simulink model "sxem_79"  (R2023a)
settings: Solver=VariableStepAuto  StartTime=0.0  StopTime=40.0  RelTol=1e-3
settings Model: Creator=User  LastModifiedBy=User

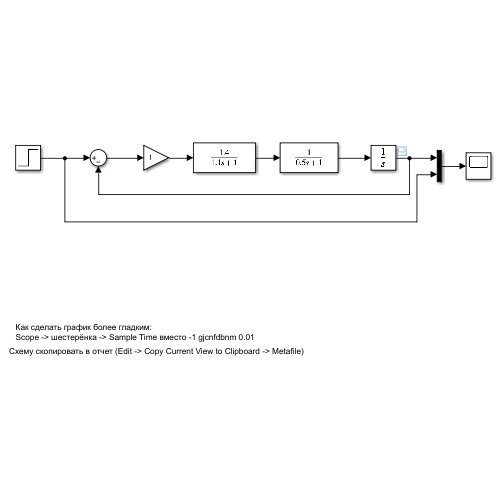
[thumbnail: Simulink's stored preview of the top-level diagram]
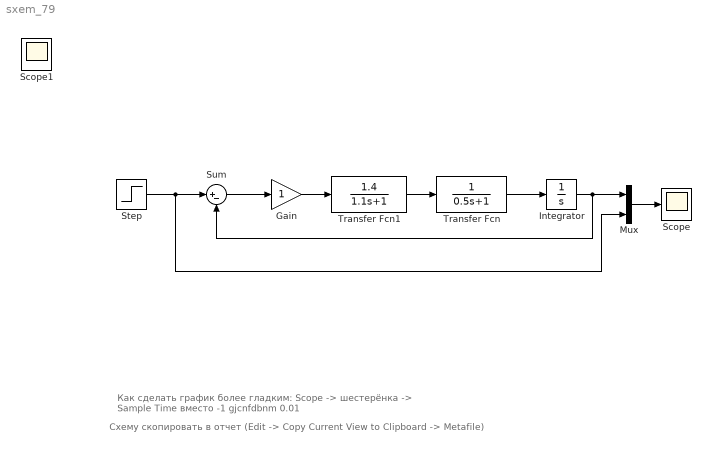
== system sxem_79 ==
  note: Как сделать график более гладким:
      | Scope -> шестерёнка -> Sample Time вместо -1 gjcnfdbnm 0.01
  note: Схему скопировать в отчет (Edit -> Copy Current View to Clipboard -> Metafile)
  Gain : Gain
  Integrator : Integrator
  Mux : Mux  Inputs=2
  Scope : Scope
  Step : Step  Time=0  SampleTime=0
  Sum : Sum  Inputs=|+-
  Transfer Fcn : TransferFcn  Denominator=[0.5 1]
  Transfer Fcn1 : TransferFcn  Numerator=[1.4]  Denominator=[1.1 1]
  Scope1 : Scope
  wires:
  Transfer Fcn1/1 -> Transfer Fcn/1
  Transfer Fcn/1 -> Integrator/1
  Integrator/1 -> Sum/2, Mux/1
  Gain/1 -> Transfer Fcn1/1
  Sum/1 -> Gain/1
  Step/1 -> Mux/2, Sum/1
  Mux/1 -> Scope/1
